simulink subsystem "APReglerA_Vorsteuerung_avRegler"  (R2020a)
settings: Solver=VariableStepAuto  StartTime=0.0  StopTime=10.0  RelTol=1e-3
model mask{AP=simparams.AP, RegData=simparams.APRegDataA, K_p_v=[], vorst_c=on, vorst_d=on}
  mask prompts: AP "Arbeitspunkt"; RegData "APRegDataA"; K_p_v "a/v-Regler Kpv"; vorst_c "Vorsteuerung Coulomb Reibung"; vorst_d "Vorsteuerung Viskose Reibung"
settings Model: Creator=Tobias  LastModifiedBy=Tobias

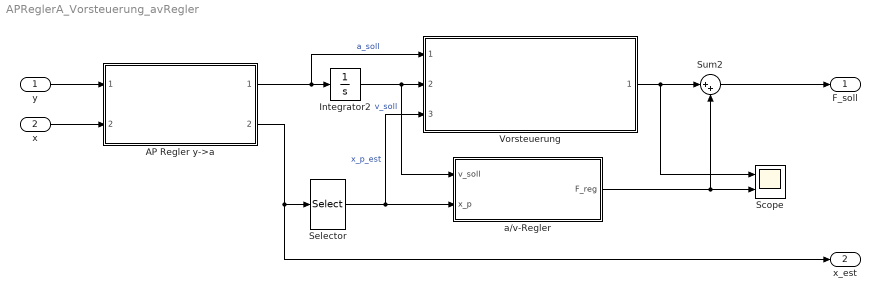
== system APReglerA_Vorsteuerung_avRegler ==
  y : Inport
  x : Inport  Port=2
  AP Regler y->a : Subsystem  ReferencedSubsystem=APRegler  AP=AP  RegData=RegData
  Integrator2 : Integrator
  Scope : Scope  NumInputPorts=2
  Selector : Selector  InputPortWidth=6  IndexOptions=Index vector (dialog)  Indices=[2]  OutputSizes=1
  Sum2 : Sum  Inputs=|++
  Vorsteuerung : Subsystem  ReferencedSubsystem=VorsteuerungSchlitten  SP=simparams.gesamtmodell.schlittenpendel  vorst=simparams.vorst
  a/v-Regler : Subsystem
  F_soll : Outport
  x_est : Outport  Port=2
  wires:
  y/1 -> AP Regler y->a/1
  x/1 -> AP Regler y->a/2
  Selector/1 -> a/v-Regler/2(x_p), Vorsteuerung/3  "x_p_est"
  Integrator2/1 -> a/v-Regler/1(v_soll), Vorsteuerung/2  "v_soll"
  AP Regler y->a/1 -> Integrator2/1, Vorsteuerung/1  "a_soll"
  Sum2/1 -> F_soll/1
  Vorsteuerung/1 -> Scope/1, Sum2/1
  AP Regler y->a/2 -> Selector/1, x_est/1
  a/v-Regler/1(F_reg) -> Scope/2, Sum2/2

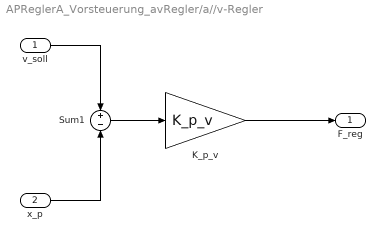
== system APReglerA_Vorsteuerung_avRegler/a//v-Regler ==
  v_soll : Inport
  x_p : Inport  Port=2
  K_p_v : Gain  Gain=K_p_v
  Sum1 : Sum  Inputs=+|-
  F_reg : Outport
  wires:
  Sum1/1 -> K_p_v/1
  x_p/1 -> Sum1/2
  v_soll/1 -> Sum1/1
  K_p_v/1 -> F_reg/1
